simulink model "iddemo_engine"  (R2015b)
settings: Solver=FixedStepDiscrete  StartTime=0.0  StopTime=20000  FixedStep=1  MaxStep=1  RelTol=1e-3
model workspace (MAT data in the model file):
  Adist = -0.7
  N = 2000
  Tdist = 200
  Ts = 0.003
  p = [-7.82997288351e-05; 0.181210895977; -0.072497134344; 0.000486358314052; 0.0361674637937]
libraries: slident x3
settings Model: Creator=The MathWorks, Inc.  LastModifiedBy=gmiglio
settings DataIOCC: SaveFormat=Array
settings DebuggingCC: SolverPrmCheckMsg=warning
settings HardwareCC: ProdBitPerPointer=32  ProdLargestAtomicFloat=None  ProdIntDivRoundTo=Undefined  ProdEndianess=Unspecified  ProdWordSize=32  ProdHWDeviceType=32-bit Generic
settings SFSimCC: SimGenImportedTypeDefs=on
settings GRTTargetCC: GeneratePreprocessorConditionals=Disable all
settings ConfigComp: CovModelRefEnable=Off  CovSFcnEnable=off

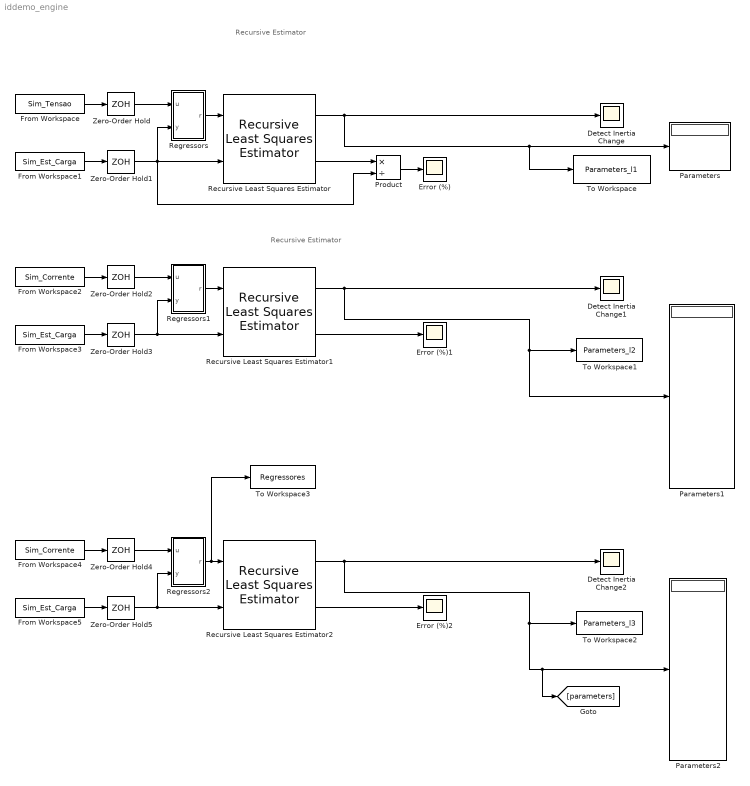
== system iddemo_engine ==
  note: Recursive Estimator
  note: Recursive Estimator
  Detect Inertia Change : Scope
  Detect Inertia Change1 : Scope
  Detect Inertia Change2 : Scope
  Error (%) : Scope
  Error (%)1 : Scope
  Error (%)2 : Scope
  From Workspace : FromWorkspace  VariableName=Sim_Tensao  SampleTime=0
  From Workspace1 : FromWorkspace  VariableName=Sim_Est_Carga  SampleTime=0
  From Workspace2 : FromWorkspace  VariableName=Sim_Corrente  SampleTime=0
  From Workspace3 : FromWorkspace  VariableName=Sim_Est_Carga  SampleTime=0
  From Workspace4 : FromWorkspace  VariableName=Sim_Corrente  SampleTime=0
  From Workspace5 : FromWorkspace  VariableName=Sim_Est_Carga  SampleTime=0
  Parameters : Display
  Parameters1 : Display
      settings: Decimation=4
  Parameters2 : Display
      settings: Decimation=4
  Product : Product  Inputs=*/
  Recursive Least Squares Estimator : slident/Estimators/Recursive Least Squares Estimator  InitialEstimateSource=None  InitialParameterData=3  P0=1  EstimationMethod=Forgetting Factor  AdaptationParameter=1-2e-4  NormalizationBias=eps  OutputError=on  OutputP=off  AddEnablePort=off  Ts=1
  Recursive Least Squares Estimator1 : slident/Estimators/Recursive Least Squares Estimator  InitialEstimateSource=None  InitialParameterData=15  P0=1  EstimationMethod=Forgetting Factor  AdaptationParameter=1-2e-4  NormalizationBias=eps  OutputError=on  OutputP=off  AddEnablePort=off  Ts=1
  Recursive Least Squares Estimator2 : slident/Estimators/Recursive Least Squares Estimator  InitialEstimateSource=None  InitialParameterData=15  P0=1  EstimationMethod=Forgetting Factor  AdaptationParameter=1-2e-4  NormalizationBias=eps  OutputError=on  OutputP=off  AddEnablePort=off  Ts=1
  Regressors : Subsystem
  Regressors1 : Subsystem
  Regressors2 : Subsystem
  To Workspace : ToWorkspace  VariableName=Parameters_l1  SaveFormat=Timeseries  SampleTime=-1
      settings: Decimation=3
  To Workspace1 : ToWorkspace  VariableName=Parameters_l2  SaveFormat=Timeseries  SampleTime=-1
      settings: Decimation=3
  To Workspace2 : ToWorkspace  VariableName=Parameters_l3  SaveFormat=Timeseries  SampleTime=-1
  To Workspace3 : ToWorkspace  VariableName=Regressores  SaveFormat=Timeseries  SampleTime=-1
  Zero-Order Hold{,1..5} (6 alike) : ZeroOrderHold
  wires:
  Regressors/1(r) -> Recursive Least Squares Estimator/1
  Recursive Least Squares Estimator/2 -> Product/1
  Product/1 -> Error (%)/1
  Recursive Least Squares Estimator/1 -> Detect Inertia Change/1, To Workspace/1, Parameters/1
  From Workspace1/1 -> Zero-Order Hold1/1
  Zero-Order Hold/1 -> Regressors/1(u)
  Zero-Order Hold1/1 -> Recursive Least Squares Estimator/2, Regressors/2(y), Product/2
  Regressors1/1(r) -> Recursive Least Squares Estimator1/1
  Recursive Least Squares Estimator1/2 -> Error (%)1/1
  Recursive Least Squares Estimator1/1 -> Detect Inertia Change1/1, To Workspace1/1, Parameters1/1
  From Workspace2/1 -> Zero-Order Hold2/1
  From Workspace3/1 -> Zero-Order Hold3/1
  Zero-Order Hold2/1 -> Regressors1/1(u)
  Zero-Order Hold3/1 -> Recursive Least Squares Estimator1/2, Regressors1/2(y)
  Regressors2/1(r) -> To Workspace3/1, Recursive Least Squares Estimator2/1
  Recursive Least Squares Estimator2/2 -> Error (%)2/1
  Recursive Least Squares Estimator2/1 -> Detect Inertia Change2/1, To Workspace2/1, [parameters], Parameters2/1
  From Workspace4/1 -> Zero-Order Hold4/1
  From Workspace5/1 -> Zero-Order Hold5/1
  Zero-Order Hold4/1 -> Regressors2/1(u)
  Zero-Order Hold5/1 -> Recursive Least Squares Estimator2/2, Regressors2/2(y)
  From Workspace/1 -> Zero-Order Hold/1

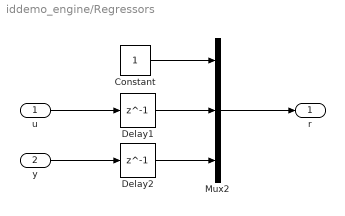
== system iddemo_engine/Regressors ==
  u : Inport
  y : Inport  Port=2
  Constant : Constant
  Delay1 : Delay  DelayLength=1  InitialCondition=1
  Delay2 : Delay  DelayLength=1  InitialCondition=2
  Mux2 : Mux  Inputs=3
  r : Outport
  wires:
  u/1 -> Delay1/1
  Mux2/1 -> r/1
  Delay1/1 -> Mux2/2
  y/1 -> Delay2/1
  Delay2/1 -> Mux2/3
  Constant/1 -> Mux2/1

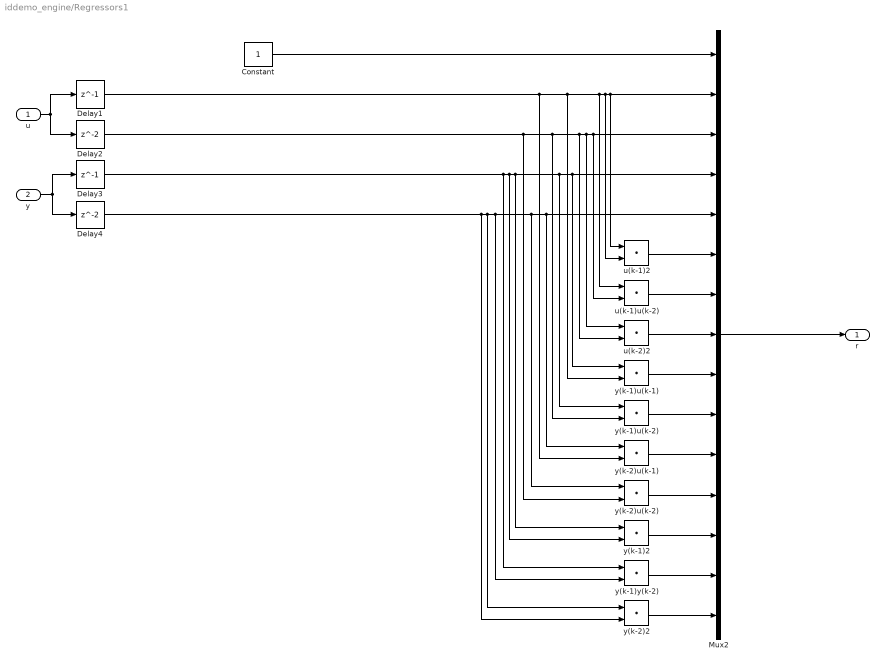
== system iddemo_engine/Regressors1 ==
  u : Inport
  y : Inport  Port=2
  Constant : Constant
  Delay1 : Delay  DelayLength=1  InitialCondition=0
  Delay2 : Delay  InitialCondition=0
  Delay3 : Delay  DelayLength=1  InitialCondition=0
  Delay4 : Delay  InitialCondition=0
  Mux2 : Mux  Inputs=15
  u(k-1)2 : DotProduct  InputSameDT=on  OutDataTypeStr=Inherit: Inherit via internal rule
  u(k-1)u(k-2) : DotProduct  InputSameDT=on  OutDataTypeStr=Inherit: Inherit via internal rule
  u(k-2)2 : DotProduct  InputSameDT=on  OutDataTypeStr=Inherit: Inherit via internal rule
  y(k-1)2 : DotProduct  InputSameDT=on  OutDataTypeStr=Inherit: Inherit via internal rule
  y(k-1)u(k-1) : DotProduct  InputSameDT=on  OutDataTypeStr=Inherit: Inherit via internal rule
  y(k-1)u(k-2) : DotProduct  InputSameDT=on  OutDataTypeStr=Inherit: Inherit via internal rule
  y(k-1)y(k-2) : DotProduct  InputSameDT=on  OutDataTypeStr=Inherit: Inherit via internal rule
  y(k-2)2 : DotProduct  InputSameDT=on  OutDataTypeStr=Inherit: Inherit via internal rule
  y(k-2)u(k-1) : DotProduct  InputSameDT=on  OutDataTypeStr=Inherit: Inherit via internal rule
  y(k-2)u(k-2) : DotProduct  InputSameDT=on  OutDataTypeStr=Inherit: Inherit via internal rule
  r : Outport
  wires:
  u/1 -> Delay1/1, Delay2/1
  Mux2/1 -> r/1
  Delay1/1 -> y(k-2)u(k-1)/2, y(k-1)u(k-1)/2, u(k-1)u(k-2)/1, u(k-1)2/2, u(k-1)2/1, Mux2/2
  Delay2/1 -> y(k-2)u(k-2)/2, y(k-1)u(k-2)/2, u(k-2)2/2, u(k-2)2/1, u(k-1)u(k-2)/2, Mux2/3
  Constant/1 -> Mux2/1
  u(k-1)2/1 -> Mux2/6
  Delay3/1 -> y(k-1)y(k-2)/1, y(k-1)2/2, y(k-1)2/1, y(k-1)u(k-2)/1, y(k-1)u(k-1)/1, Mux2/4
  Delay4/1 -> y(k-2)2/2, y(k-2)2/1, y(k-1)y(k-2)/2, y(k-2)u(k-2)/1, y(k-2)u(k-1)/1, Mux2/5
  y/1 -> Delay3/1, Delay4/1
  u(k-1)u(k-2)/1 -> Mux2/7
  u(k-2)2/1 -> Mux2/8
  y(k-1)u(k-1)/1 -> Mux2/9
  y(k-1)u(k-2)/1 -> Mux2/10
  y(k-2)u(k-1)/1 -> Mux2/11
  y(k-2)u(k-2)/1 -> Mux2/12
  y(k-1)2/1 -> Mux2/13
  y(k-1)y(k-2)/1 -> Mux2/14
  y(k-2)2/1 -> Mux2/15

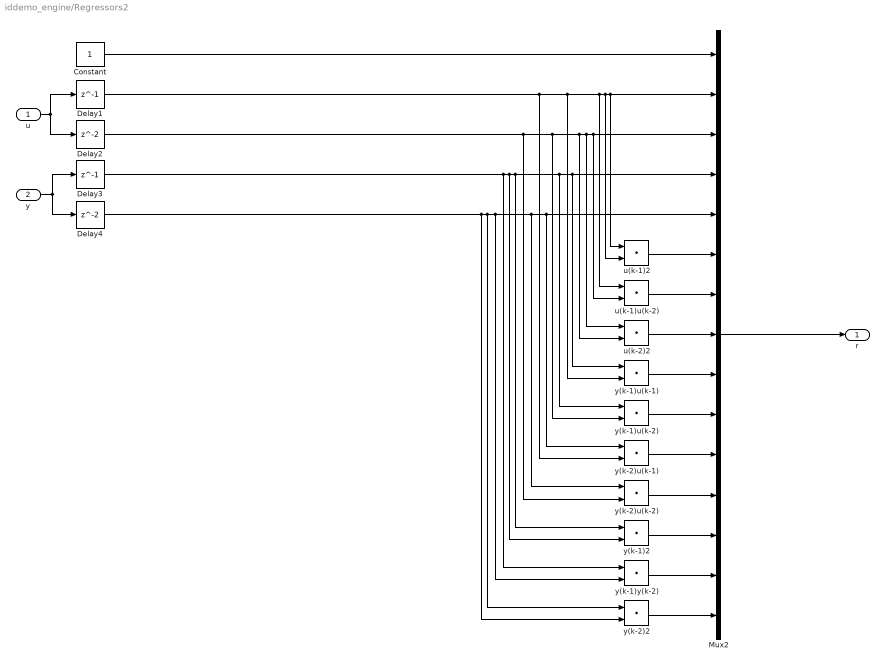
== system iddemo_engine/Regressors2 ==
  u : Inport
  y : Inport  Port=2
  Constant : Constant
  Delay1 : Delay  DelayLength=1  InitialCondition=0
  Delay2 : Delay  InitialCondition=0
  Delay3 : Delay  DelayLength=1  InitialCondition=0
  Delay4 : Delay  InitialCondition=0
  Mux2 : Mux  Inputs=15
  u(k-1)2 : DotProduct  InputSameDT=on  OutDataTypeStr=Inherit: Inherit via internal rule
  u(k-1)u(k-2) : DotProduct  InputSameDT=on  OutDataTypeStr=Inherit: Inherit via internal rule
  u(k-2)2 : DotProduct  InputSameDT=on  OutDataTypeStr=Inherit: Inherit via internal rule
  y(k-1)2 : DotProduct  InputSameDT=on  OutDataTypeStr=Inherit: Inherit via internal rule
  y(k-1)u(k-1) : DotProduct  InputSameDT=on  OutDataTypeStr=Inherit: Inherit via internal rule
  y(k-1)u(k-2) : DotProduct  InputSameDT=on  OutDataTypeStr=Inherit: Inherit via internal rule
  y(k-1)y(k-2) : DotProduct  InputSameDT=on  OutDataTypeStr=Inherit: Inherit via internal rule
  y(k-2)2 : DotProduct  InputSameDT=on  OutDataTypeStr=Inherit: Inherit via internal rule
  y(k-2)u(k-1) : DotProduct  InputSameDT=on  OutDataTypeStr=Inherit: Inherit via internal rule
  y(k-2)u(k-2) : DotProduct  InputSameDT=on  OutDataTypeStr=Inherit: Inherit via internal rule
  r : Outport
  wires:
  u/1 -> Delay1/1, Delay2/1
  Mux2/1 -> r/1
  Delay1/1 -> y(k-2)u(k-1)/2, y(k-1)u(k-1)/2, u(k-1)u(k-2)/1, u(k-1)2/2, u(k-1)2/1, Mux2/2
  Delay2/1 -> y(k-2)u(k-2)/2, y(k-1)u(k-2)/2, u(k-2)2/2, u(k-2)2/1, u(k-1)u(k-2)/2, Mux2/3
  Constant/1 -> Mux2/1
  u(k-1)2/1 -> Mux2/6
  Delay3/1 -> y(k-1)y(k-2)/1, y(k-1)2/2, y(k-1)2/1, y(k-1)u(k-2)/1, y(k-1)u(k-1)/1, Mux2/4
  Delay4/1 -> y(k-2)2/2, y(k-2)2/1, y(k-1)y(k-2)/2, y(k-2)u(k-2)/1, y(k-2)u(k-1)/1, Mux2/5
  y/1 -> Delay3/1, Delay4/1
  u(k-1)u(k-2)/1 -> Mux2/7
  u(k-2)2/1 -> Mux2/8
  y(k-1)u(k-1)/1 -> Mux2/9
  y(k-1)u(k-2)/1 -> Mux2/10
  y(k-2)u(k-1)/1 -> Mux2/11
  y(k-2)u(k-2)/1 -> Mux2/12
  y(k-1)2/1 -> Mux2/13
  y(k-1)y(k-2)/1 -> Mux2/14
  y(k-2)2/1 -> Mux2/15
